simulink model "viv"  (R2020a)
settings: Solver=VariableStepAuto  StartTime=0.0  StopTime=120.0  RelTol=1e-3
values from neighbouring files (symbols this model uses):
  c = 4*pi*0.99*0.031    (= 0.385661914155)    [VIV_params.m]
  C_f = 1.5    [VIV_params.m]
  k = 245    [VIV_params.m]
  m = 2    [VIV_params.m]
  rho = 800    [VIV_params.m]
settings Model: Creator=Sumit  LastModifiedBy=Sumit

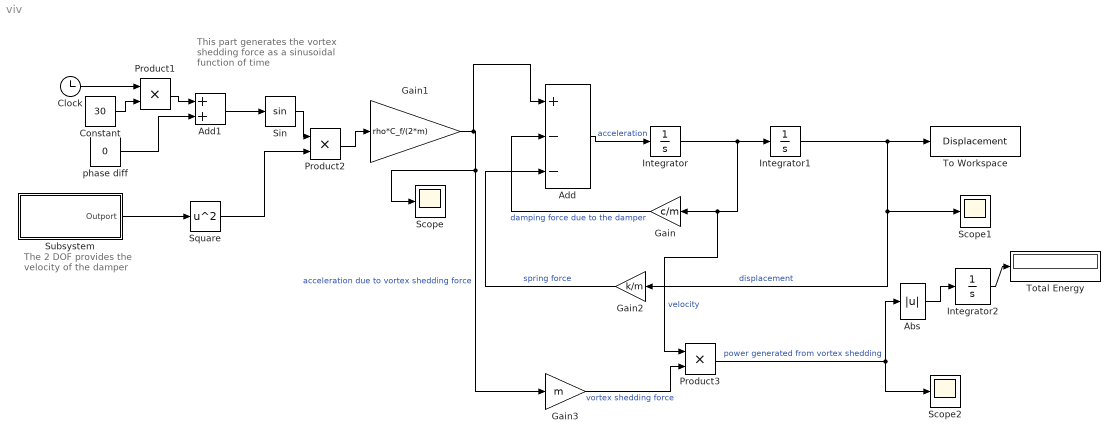
== system viv ==
  note: The 2 DOF provides the velocity of the damper
  note: This part generates the vortex shedding force as a sinusoidal function of time
  Abs : Abs
  Add : Sum  Inputs=+--
  Add1 : Sum
  Clock : Clock
  Constant : Constant  Value=30
  Gain : Gain  Gain=c/m
  Gain1 : Gain  Gain=rho*C_f/(2*m)
  Gain2 : Gain  Gain=k/m
  Gain3 : Gain  Gain=m
  Integrator : Integrator
  Integrator1 : Integrator
  Integrator2 : Integrator
  Product1 : Product
  Product2 : Product
  Product3 : Product
  Scope : Scope
  Scope1 : Scope
  Scope2 : Scope
  Sin : Trigonometry
  Square : Math  Operator=square  SaturateOnIntegerOverflow=on
  Subsystem : Subsystem
  To Workspace : ToWorkspace  VariableName=Displacement  SaveFormat=Timeseries  SampleTime=-1
  Total Energy : Display
  phase diff : Constant  Value=0
  wires:
  Gain1/1 -> Add/1, Gain3/1, Scope/1  "acceleration due to vortex shedding force"
  Add/1 -> Integrator/1  "acceleration"
  Integrator/1 -> Integrator1/1, Product3/1, Gain/1  "velocity"
  Gain/1 -> Add/2  "damping force due to the damper"
  Integrator1/1 -> Scope1/1, Gain2/1, To Workspace/1  "displacement"
  Gain2/1 -> Add/3  "spring force"
  Clock/1 -> Product1/1
  Constant/1 -> Product1/2
  Product1/1 -> Add1/1
  phase diff/1 -> Add1/2
  Add1/1 -> Sin/1
  Subsystem/1(Outport) -> Square/1
  Sin/1 -> Product2/1
  Square/1 -> Product2/2
  Product2/1 -> Gain1/1
  Gain3/1 -> Product3/2  "vortex shedding force"
  Product3/1 -> Abs/1, Scope2/1  "power generated from vortex shedding"
  Integrator2/1 -> Total Energy/1
  Abs/1 -> Integrator2/1

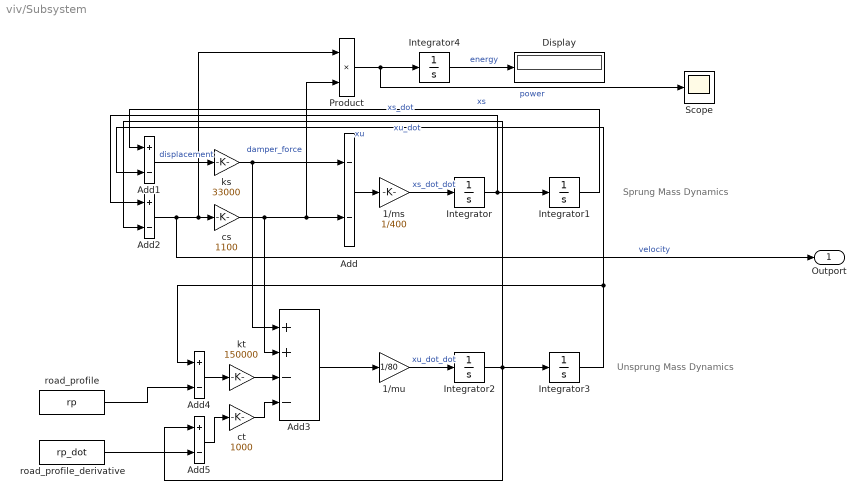
== system viv/Subsystem ==
  note: Sprung Mass Dynamics
  note: Unsprung Mass Dynamics
  1/ms : Gain  Gain=1/400
  1/mu : Gain  Gain=1/80
  Add : Sum  Inputs=--
  Add{1..2,4..5} (4 alike) : Sum  Inputs=+-
  Add3 : Sum  Inputs=++--
  Display : Display
      settings: Decimation=2
  Integrator{,1..4} (5 alike) : Integrator
  Product : Product
  Scope : Scope
  cs : Gain  Gain=1100
  ct : Gain  Gain=1000
  ks : Gain  Gain=33000
  kt : Gain  Gain=150000
  road_profile : FromWorkspace  VariableName=rp
  road_profile_derivative : FromWorkspace  VariableName=rp_dot
  Outport : Outport
  wires:
  cs/1 -> Add3/2, Add/2, Product/2  "damper_force"
  Product/1 -> Scope/1, Integrator4/1  "power"
  kt/1 -> Add3/3
  Integrator4/1 -> Display/1  "energy"
  Integrator/1 -> Integrator1/1, Add2/1  "xs_dot"
  Add2/1 -> Outport/1, Product/1, cs/1  "velocity"
  Integrator1/1 -> Add1/1  "xs"
  Add1/1 -> ks/1  "displacement"
  Add/1 -> 1/ms/1
  ct/1 -> Add3/4
  ks/1 -> Add3/1, Add/1
  Add3/1 -> 1/mu/1
  road_profile/1 -> Add4/2
  Integrator3/1 -> Add1/2, Add4/1  "xu"
  Integrator2/1 -> Add5/1, Add2/2, Integrator3/1  "xu_dot"
  Add4/1 -> kt/1
  road_profile_derivative/1 -> Add5/2
  1/mu/1 -> Integrator2/1  "xu_dot_dot"
  1/ms/1 -> Integrator/1  "xs_dot_dot"
  Add5/1 -> ct/1
